simulink model "Test_Logic_Operation_Bitwise_XOR"  (Simulink 8.1)
settings: Solver=VariableStepDiscrete  StartTime=0.0  StopTime=len  RelTol=1e-3
libraries: Logic_Operations_Lib x1
settings Model: Creator=uzivatel  LastModifiedBy=uzivatel
settings DataIOCC: SignalLoggingSaveFormat=Dataset
settings OptimizationCC: ExpressionDepthLimit=128
settings DebuggingCC: FcnCallInpInsideContextMsg=EnableAllAsError
settings GRTTargetCC: CombineOutputUpdateFcns=on  GRTInterface=off

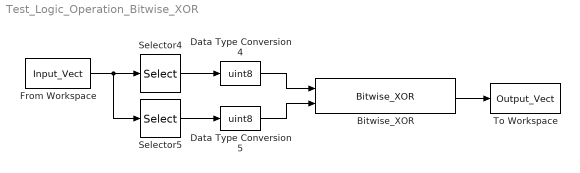
== system Test_Logic_Operation_Bitwise_XOR ==
  Bitwise_XOR : Logic_Operations_Lib/Logic_Operations_Lib/Bitwise_XOR
  Data Type Conversion4 : DataTypeConversion  OutDataTypeStr=uint8
  Data Type Conversion5 : DataTypeConversion  OutDataTypeStr=uint8
  From Workspace : FromWorkspace  VariableName=Input_Vect  SampleTime=1  Interpolate=off  OutputAfterFinalValue=Holding final value
  Selector4 : Selector  IndexMode=Zero-based  InputPortWidth=2  SampleTime=1  IndexOptions=Index vector (dialog)  Indices=0  OutputSizes=1
  Selector5 : Selector  IndexMode=Zero-based  InputPortWidth=2  SampleTime=1  IndexOptions=Index vector (dialog)  Indices=1  OutputSizes=1
  To Workspace : ToWorkspace  VariableName=Output_Vect  SampleTime=1
  wires:
  Bitwise_XOR/1 -> To Workspace/1
  Data Type Conversion5/1 -> Bitwise_XOR/2
  Data Type Conversion4/1 -> Bitwise_XOR/1
  From Workspace/1 -> Selector5/1, Selector4/1
  Selector4/1 -> Data Type Conversion4/1
  Selector5/1 -> Data Type Conversion5/1
